simulink model "Feedforward"  (R2019a)
settings: Solver=VariableStepAuto  StartTime=0.0  StopTime=20  RelTol=1e-3
settings Model: Creator=Usuario  LastModifiedBy=Usuario

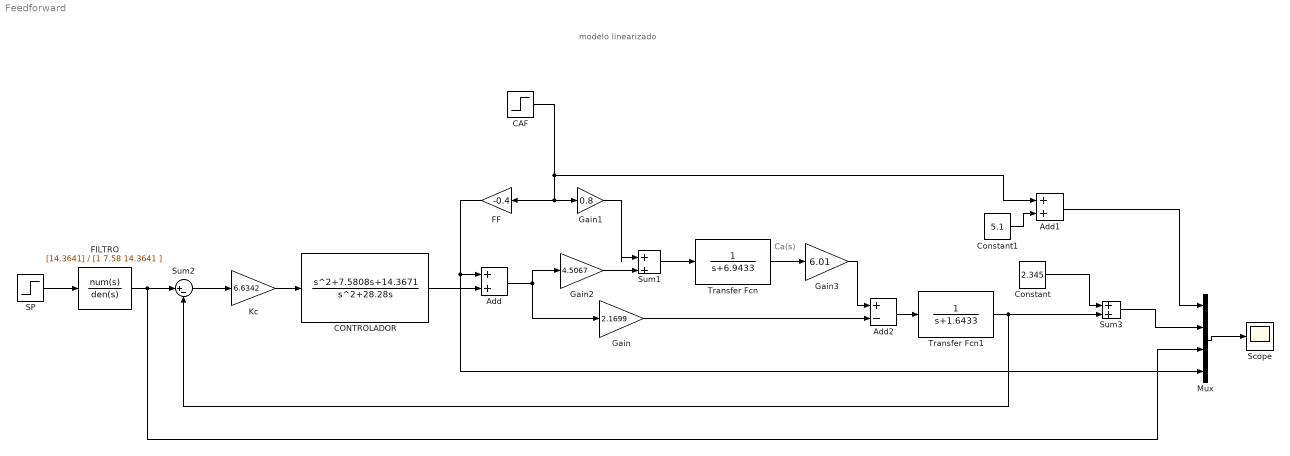
== system Feedforward ==
  note: Ca(s)
  note: modelo linearizado
  Add : Sum
  Add1 : Sum
  Add2 : Sum  Inputs=+-
  CAF : Step  Time=10  After=0.1  SampleTime=0.01
  "CONTROLADOR " : TransferFcn  Numerator=[1 7.5808 14.3671]  Denominator=[1 28.28 0]
  Constant : Constant  Value=2.345
  Constant1 : Constant  Value=5.1
  FF : Gain  Gain=-0.4
  "FILTRO " : TransferFcn  Numerator=[14.3641]  Denominator=[1 7.58 14.3641 ]
  Gain : Gain  Gain=2.1699
  Gain1 : Gain  Gain=0.8
  Gain2 : Gain  Gain=4.5067
  Gain3 : Gain  Gain=6.01
  "Kc " : Gain  Gain=6.6342
  Mux : Mux
  SP : Step  Time=5  After=0.1  SampleTime=0.01
  Scope : Scope
  Sum1 : Sum  Inputs=|++
  Sum2 : Sum  Inputs=|+-
  Sum3 : Sum  Inputs=|++
  Transfer Fcn : TransferFcn  Denominator=[1 6.9433]
  Transfer Fcn1 : TransferFcn  Denominator=[1 1.6433]
  wires:
  Add2/1 -> Transfer Fcn1/1
  Gain1/1 -> Sum1/1
  Gain2/1 -> Sum1/2
  Sum1/1 -> Transfer Fcn/1
  "Kc "/1 -> "CONTROLADOR "/1
  CAF/1 -> Gain1/1, FF/1, Add1/1
  Sum2/1 -> "Kc "/1
  Transfer Fcn1/1 -> Sum2/2, Sum3/2
  "FILTRO "/1 -> Mux/3, Sum2/1
  Mux/1 -> Scope/1
  SP/1 -> "FILTRO "/1
  Constant/1 -> Sum3/1
  Sum3/1 -> Mux/2
  "CONTROLADOR "/1 -> Add/2
  Add/1 -> Gain/1, Gain2/1
  Constant1/1 -> Add1/2
  Add1/1 -> Mux/1
  FF/1 -> Mux/4, Add/1
  Transfer Fcn/1 -> Gain3/1
  Gain3/1 -> Add2/1
  Gain/1 -> Add2/2
